simulink model "linearModelMatrix"  (R2014b)
settings: Solver=ode4  StartTime=0.0  StopTime=TIME_SIM  FixedStep=STEP_SIZE  RelTol=1e-3
values from neighbouring files (symbols this model uses):
  C = [0 0 1]    [mainbis.m]
undefined symbols (not defined in the file or in its folder): A, B
settings Model: Creator=Kate  LastModifiedBy=Kate
settings DataIOCC: SaveState=on

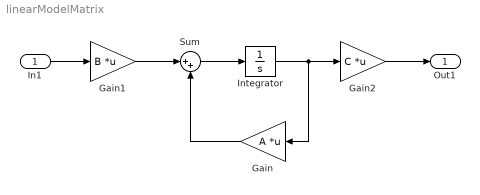
== system linearModelMatrix ==
  In1 : Inport
  Gain : Gain  Gain=A  Multiplication=Matrix(K*u)
  Gain1 : Gain  Gain=B  Multiplication=Matrix(K*u)
  Gain2 : Gain  Gain=C  Multiplication=Matrix(K*u)
  Integrator : Integrator
  Sum : Sum  Inputs=|++
  Out1 : Outport
  wires:
  Sum/1 -> Integrator/1
  Integrator/1 -> Gain2/1, Gain/1
  Gain/1 -> Sum/2
  Gain1/1 -> Sum/1
  In1/1 -> Gain1/1
  Gain2/1 -> Out1/1
